simulink model "PWM_car"  (R2018a)
settings: Solver=VariableStepAuto  StartTime=0.0  StopTime=10.0  RelTol=1e-3
settings Model: Creator=shami  LastModifiedBy=shami

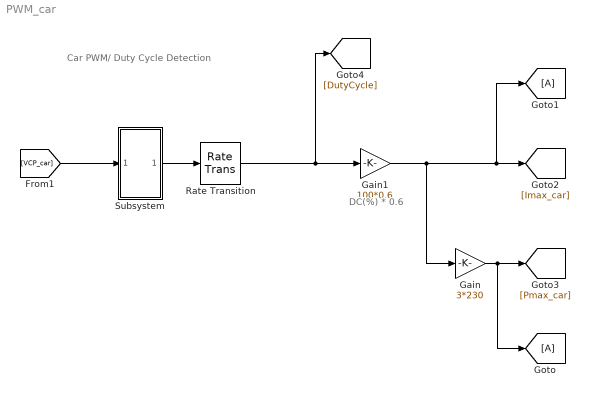
== system PWM_car ==
  note: DC(%) * 0.6
  note: Car PWM/ Duty Cycle Detection
  Gain : Gain  Gain=3*230
  Gain1 : Gain  Gain=100*0.6
  Rate Transition : RateTransition
  Subsystem : Subsystem
  wires:
  Gain/1 -> [Pmax_car], [A]
  Gain1/1 -> [A], [Imax_car], Gain/1
  [VCP_car] -> Subsystem/1(pwm)
  Subsystem/1(Out1) -> Rate Transition/1
  Rate Transition/1 -> [DutyCycle], Gain1/1

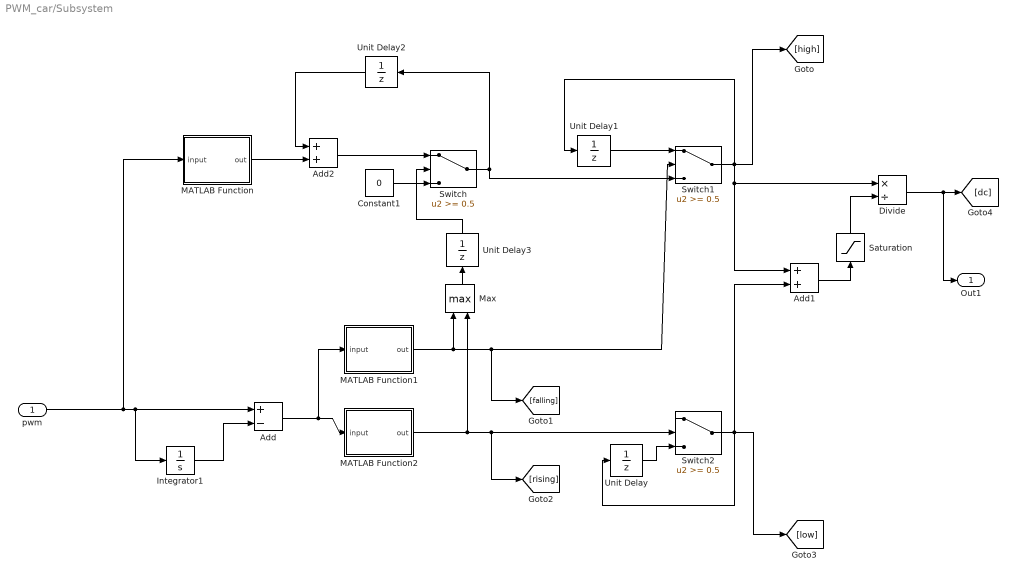
== system PWM_car/Subsystem ==
  pwm : Inport
  Add : Sum  Inputs=+-
  Add1 : Sum
  Add2 : Sum
  Constant1 : Constant  Value=0
  Divide : Product  Inputs=*/
  Integrator1 : Integrator
  MATLAB Function : MATLAB Function  TreatAsAtomicUnit=on
  MATLAB Function1 : MATLAB Function  TreatAsAtomicUnit=on
  MATLAB Function2 : MATLAB Function  TreatAsAtomicUnit=on
  Max : MinMax  Function=max  Inputs=2
  Saturation : Saturate  UpperLimit=inf  LowerLimit=1e-5
  Switch : Switch  Threshold=0.5
  Switch1 : Switch  Threshold=0.5
  Switch2 : Switch  Threshold=0.5
  Unit Delay{,1..3} (4 alike) : UnitDelay  SampleTime=-1
  Out1 : Outport
  wires:
  Integrator1/1 -> Add/2
  pwm/1 -> MATLAB Function/1(input), Add/1, Integrator1/1
  Constant1/1 -> Switch/3
  Switch/1 -> Unit Delay2/1, Switch1/3
  Max/1 -> Unit Delay3/1
  Unit Delay1/1 -> Switch1/1
  Switch1/1 -> Unit Delay1/1, [high], Add1/1, Divide/1
  Unit Delay3/1 -> Switch/2
  MATLAB Function1/1(out) -> Switch1/2, [falling], Max/1
  MATLAB Function2/1(out) -> Max/2, [rising], Switch2/2
  Switch2/1 -> Unit Delay/1, [low], Add1/2
  Unit Delay/1 -> Switch2/3
  Add1/1 -> Saturation/1
  Saturation/1 -> Divide/2
  Divide/1 -> Out1/1, [dc]
  Unit Delay2/1 -> Add2/1
  MATLAB Function/1(out) -> Add2/2
  Add2/1 -> Switch/1
  Add/1 -> MATLAB Function1/1(input), MATLAB Function2/1(input)

== matlab function PWM_car/Subsystem/MATLAB Function1 ==
  data: input input; out output
function out = fcn(input)
int temp = 0;
if(input > -1)
    y = 1;
    int temp = y ; 
    
elseif (input < -1)
    y = 0; 
    int temp = y ; 
    
elseif (input == -1)
    y = temp ;
      
end

out = y;

== matlab function PWM_car/Subsystem/MATLAB Function ==
  data: input input; out output
function out = fcn(input)
int temp = 0;
if(input > -1000)
    y = 1;
    int temp = y ; 
    
elseif (input < -1000)
    y = 0; 
    int temp = y ; 
    
elseif (input == -1000)
    y = temp ;
      
end

out = y;

== matlab function PWM_car/Subsystem/MATLAB Function2 ==
  data: input input; out output
function out = fcn(input)
int temp = 0;
if(input > 1)
    y = 1;
    int temp = y ; 
    
elseif (input < 1)
    y = 0; 
    int temp = y ; 
    
elseif (input == 1)
    y = temp ;
      
end

out = y;
